simulink model "GFLIB_Hyst_BAM"  (Simulink 9.3)
settings: Solver=VariableStepAuto  StartTime=0.0  StopTime=10.0  RelTol=1e-3
settings Model: Creator=nxa18952  LastModifiedBy=nxa18952
settings DataIOCC: SaveFormat=Dataset  SignalLoggingSaveFormat=Dataset  ReturnWorkspaceOutputs=on
settings OptimizationCC: LifeSpan=auto
settings DebuggingCC: UnderspecifiedInitializationDetection=Simplified  MergeDetectMultiDrivingBlocksExec=error  FcnCallInpInsideContextMsg=error  SFUnexpectedBacktrackingDiag=error  SFNoUnconditionalDefaultTransitionDiag=error  SFExecutionAtInitializationDiag=warning  ArithmeticOperatorsInVariantConditions=error
settings HardwareCC: ProdBitPerPointer=64  ProdBitPerSizeT=64  ProdBitPerPtrDiffT=64  ProdLargestAtomicFloat=Float  ProdIntDivRoundTo=Zero  ProdEndianess=LittleEndian  ProdWordSize=64  ProdHWDeviceType=Intel->x86-64 (Windows64)
settings ModelReferenceCC: PropagateSignalLabelsOutOfModel=on
settings SFSimCC: SimUseLocalCustomCode=on
settings RTWCC: RTWUseLocalCustomCode=on
settings CodeAppCC: StateflowObjectComments=off
settings GRTTargetCC: TargetLangStandard=C99 (ISO)  CombineOutputUpdateFcns=on  GRTInterface=off
settings ConfigComp: CovMetricSettings=dwe  CovHtmlReporting=off  CovSaveCumulativeToWorkspaceVar=off  CovSaveSingleToWorkspaceVar=off  CovExternalEMLEnable=on

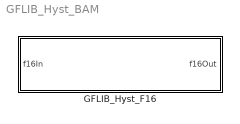
== system GFLIB_Hyst_BAM ==
  GFLIB_Hyst_F16 : Subsystem  TreatAsAtomicUnit=on  mask(GFLIB_Hyst_F16){showStates=Hide (faster execution), f16HystOn=0, f16HystOff=0, f16OutValOn=0, f16OutValOff=0}
      mask prompts: showStates "Show internal states"; f16HystOn "f16HystOn (Value determining the upper threshold)"; f16HystOff "f16HystOff (Value determining the lower threshold)"; f16OutValOn "f16OutValOn (Value of the output when input is higher than the upper threshold)"; f16OutValOff "f16OutValOff (Value of the output when input is lower than the lower threshold)"
      mask help: Hysteresis function in 16-bit fixed-point fractional implementation. Refer to the AMMCLIB User's Guide for further details.
      mask init:
      | if ~evalin('base','exist(''tS8'',''var'')')
      |   if (2 ~= exist('SWLIBS_Typedefs.mat','file'))
      |       error('File SWLIBS_Typedefs.mat is not on the Matlab path. Please add the AMMCLIB "bam" folder in the Matlab Search Path.');
      |   else
      |       evalin('base', 'load(''SWLIBS_Typedefs.mat'')');
      |   end
      | end
      | if showStates == 1
      |     % hidden state variables
      |     if strcmp(get_param([gcb '/f16HystOn'], 'BlockType'), 'Inport')
      |         posblk = get_param(gcb, 'Position');
      | 
      |         pos = get_param(    [gcb, '/f16HystOn'], 'Position');
      |         orient = get_param( [gcb, '/f16HystOn'], 'Orientation');
      |         delete_block(       [gcb, '/f16HystOn']);
      |         add_block('built-in/Ground', [gcb, '/f16HystOn'], 'Position', pos, 'Orientation', orient);
      | 
      |         pos = get_param(    [gcb, '/f16HystOff'], 'Position');
      |         orient = get_param( [gcb, '/f16HystOff'], 'Orientation');
      |         delete_block(       [gcb, '/f16HystOff']);
      |         add_block('built-in/Ground', [gcb, '/f16HystOff'], 'Position', pos, 'Orientation', orient);
      | 
      |         pos = get_param(    [gcb, '/f16OutValOn'], 'Position');
      |         orient = get_param( [gcb, '/f16OutValOn'], 'Orientation');
      |         delete_block(       [gcb, '/f16OutValOn']);
      |         add_block('built-in/Ground', [gcb, '/f16OutValOn'], 'Position', pos, 'Orientation', orient);
      | 
      |         pos = get_param(    [gcb, '/f16OutValOff'], 'Position');
      |         orient = get_param( [gcb, '/f16OutValOff'], 'Orientation');
      |         delete_block(       [gcb, '/f16OutValOff']);
      |         add_block('built-in/Ground', [gcb, '/f16OutValOff'], 'Position', pos, 'Orientation', orient);
      | 
      |         pos = get_param(    [gcb, '/f16OutState'], 'Position');
      |         orient = get_param( [gcb, '/f16OutState'], 'Orientation');
      |         delete_block(       [gcb, '/f16OutState']);
      |         add_block('built-in/Ground', [gcb, '/f16OutState'], 'Position', pos, 'Orientation', orient);
      | 
      | 
      |         pos = get_param(    [gcb '/f16OutState_Out'], 'Position');
      |         orient = get_param( [gcb '/f16OutState_Out'], 'Orientation');
      |         delete_block(       [gcb '/f16OutState_Out']);
      |         add_block('built-in/Terminator', [gcb '/f16OutState_Out'], 'Position', pos, 'Orientation', orient);
      | 
      | 
      |         set_param([gcb '/f16In'], 'Port', '1');
      | 
      |         set_param([gcb '/f16Out'], 'Port', '1');
      | 
      |         set_param(gcb,'MaskEnables',{'on','on','on','on','on'});
      | 
      |         if (posblk(4) - posblk(2)) > 50
      |           height = 50;
      |           set_param(gcb,'Position',[posblk(1), posblk(2), posblk(3), posblk(2)+height])
      |         end
      |     end
      | else
      |     % shown state variables
      |     if strcmp(get_param([gcb '/f16HystOn'], 'BlockType'), 'Ground')
      |         posblk = get_param(gcb, 'Position');
      | 
      |         pos = get_param(    [gcb, '/f16HystOn'], 'Position');
      |         orient = get_param( [gcb, '/f16HystOn'], 'Orientation');
      |         delete_block(       [gcb, '/f16HystOn']);
      |         add_block('built-in/Inport', [gcb, '/f16HystOn'], 'Position', pos, 'Orientation', orient, 'OutDataTypeStr', 'int16');
      | 
      |         pos = get_param(    [gcb, '/f16HystOff'], 'Position');
      |         orient = get_param( [gcb, '/f16HystOff'], 'Orientation');
      |         delete_block(       [gcb, '/f16HystOff']);
      |         add_block('built-in/Inport', [gcb, '/f16HystOff'], 'Position', pos, 'Orientation', orient, 'OutDataTypeStr', 'int16');
      | 
      |         pos = get_param(    [gcb, '/f16OutValOn'], 'Position');
      |         orient = get_param( [gcb, '/f16OutValOn'], 'Orientation');
      |         delete_block(       [gcb, '/f16OutValOn']);
      |         add_block('built-in/Inport', [gcb, '/f16OutValOn'], 'Position', pos, 'Orientation', orient, 'OutDataTypeStr', 'int16');
      | 
      |         pos = get_param(    [gcb, '/f16OutValOff'], 'Position');
      |         orient = get_param( [gcb, '/f16OutValOff'], 'Orientation');
      |         delete_block(       [gcb, '/f16OutValOff']);
      |         add_block('built-in/Inport', [gcb, '/f16OutValOff'], 'Position', pos, 'Orientation', orient, 'OutDataTypeStr', 'int16');
      | 
      |         pos = get_param(    [gcb, '/f16OutState'], 'Position');
      |         orient = get_param( [gcb, '/f16OutState'], 'Orientation');
      |         delete_block(       [gcb, '/f16OutState']);
      |         add_block('built-in/Inport', [gcb, '/f16OutState'], 'Position', pos, 'Orientation', orient, 'OutDataTypeStr', 'int16');
      | 
      | 
      |         pos = get_param(    [gcb '/f16OutState_Out'], 'Position');
      |         orient = get_param( [gcb '/f16OutState_Out'], 'Orientation');
      |         delete_block(       [gcb '/f16OutState_Out']);
      |         add_block('built-in/Outport', [gcb '/f16OutState_Out'], 'Position', pos, 'Orientation', orient);
      | 
      | 
      |         set_param([gcb '/f16In'], 'Port', '1');
      |         set_param([gcb '/f16HystOn'], 'Port', '2');
      |         set_param([gcb '/f16HystOff'], 'Port', '3');
      |         set_param([gcb '/f16OutValOn'], 'Port', '4');
      |         set_param([gcb '/f16OutValOff'], 'Port', '5');
      |         set_param([gcb '/f16OutState'], 'Port', '6');
      | 
      |         set_param([gcb '/f16Out'], 'Port', '1');
      |         set_param([gcb '/f16OutState_Out'], 'Port', '2');
      | 
      |         set_param(gcb,'MaskEnables',{'on','off','off','off','off'});
      | 
      |         if (posblk(4) - posblk(2)) < 175
      |           height = 175;
      |           set_param(gcb,'Position',[posblk(1), posblk(2), posblk(3), posblk(2)+height])
      |         end
      |     end
      | end
      settings: RTWSystemCode=Inline
      mask TypeOptions showStates: Hide (faster execution) | Show (allows debugging; connect feedback loops manually)
      mask Callback showStates:
      | maskStr = get_param(gcb,'showStates');
      | if strcmp(maskStr,'Hide (faster execution)'),
      |     set_param(gcb,'MaskEnables',{'on','on','on','on','on'});
      | else
      |     set_param(gcb,'MaskEnables',{'on','off','off','off','off'});
      | end
      mask Display:
      | color('black');
      | pos = get_param(gcb, 'Position');
      | width = pos(3) - pos(1);
      | height = pos(4) - pos(2);
      | tX=width/2;
      | tY=height - 8;
      | color('black');
      | text(tX,tY, 'GFLIB_Hyst_F16', 'horizontalAlignment', 'center');
      | if showStates == 2
      |   color('red');
      |   text(tX,tY - 20, ['debugging mode' char(13) char(10) '(limited performance)'], 'horizontalAlignment', 'center');
      | end

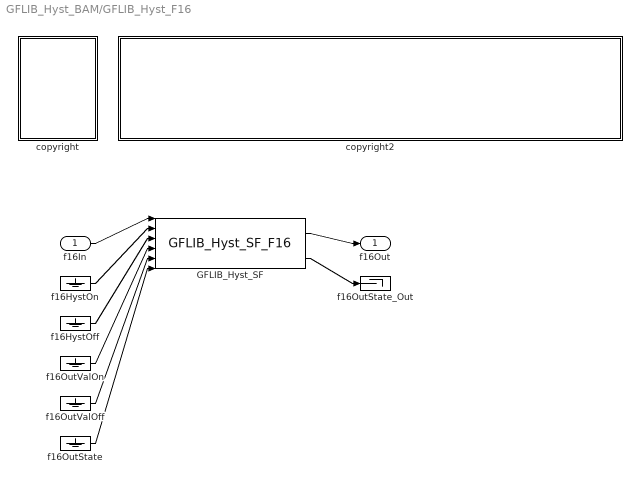
== system GFLIB_Hyst_BAM/GFLIB_Hyst_F16 ==
  f16In : Inport  OutDataTypeStr=int16
  GFLIB_Hyst_SF : S-Function  FunctionName=GFLIB_Hyst_SF_F16  Parameters=showStates,f16HystOn,f16HystOff,f16OutValOn,f16OutValOff  SFunctionDeploymentMode=off  EnableBusSupport=off
  copyright : Subsystem
      mask Display: text(10,90,'FILE:');text(10,75,'DESRIPTION:');text(10,60,'COPYRIGHT:');text(10,45,'VERSION:');text(10,30,'DATE:')
  copyright2 : Subsystem
      mask Display: text(10,90,'GFLIB_Hyst_BAM_F16.mdl');text(10,75,'Hysteresis function.');text(10,60,'NXP 2020');text(10,45,'1.0');text(10,30,'18-Mar-2020');
  f16HystOff : Ground
  f16HystOn : Ground
  f16OutState : Ground
  f16OutState_Out : Terminator
  f16OutValOff : Ground
  f16OutValOn : Ground
  f16Out : Outport
  wires:
  f16In/1 -> GFLIB_Hyst_SF/1
  f16HystOn/1 -> GFLIB_Hyst_SF/2
  f16HystOff/1 -> GFLIB_Hyst_SF/3
  f16OutValOn/1 -> GFLIB_Hyst_SF/4
  f16OutValOff/1 -> GFLIB_Hyst_SF/5
  f16OutState/1 -> GFLIB_Hyst_SF/6
  GFLIB_Hyst_SF/1 -> f16Out/1
  GFLIB_Hyst_SF/2 -> f16OutState_Out/1

== system GFLIB_Hyst_BAM/GFLIB_Hyst_F16/copyright ==

== system GFLIB_Hyst_BAM/GFLIB_Hyst_F16/copyright2 ==
